simulink subsystem "calcErrorOuterLoop"  (R2026a)
settings: Solver=VariableStepAuto
settings Model: Creator=maxhu  LastModifiedBy=maxhu

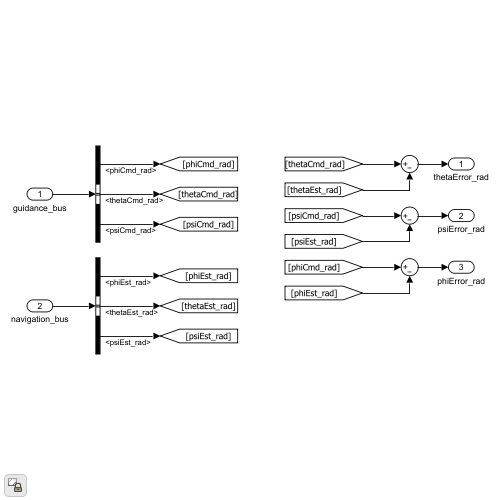
[thumbnail: Simulink's stored preview of the top-level diagram]
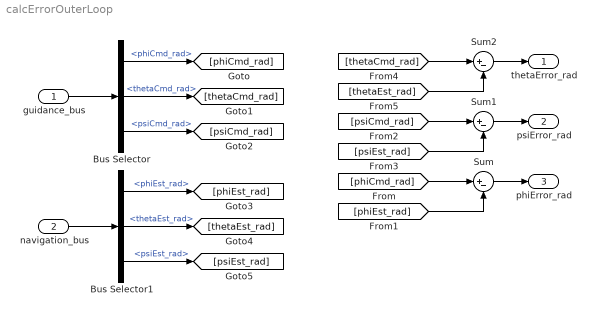
== system calcErrorOuterLoop ==
  guidance_bus : Inport
  navigation_bus : Inport  Port=2
  Bus Selector : BusSelector  OutputSignals=phiCmd_rad,thetaCmd_rad,psiCmd_rad
  Bus Selector1 : BusSelector  OutputSignals=phiEst_rad,thetaEst_rad,psiEst_rad
  Sum : Sum  Inputs=|+-
  Sum1 : Sum  Inputs=|+-
  Sum2 : Sum  Inputs=|+-
  thetaError_rad : Outport
  psiError_rad : Outport  Port=2
  phiError_rad : Outport  Port=3
  wires:
  guidance_bus/1 -> Bus Selector/1
  Bus Selector/1 -> [phiCmd_rad]  "<phiCmd_rad>"
  Bus Selector/2 -> [thetaCmd_rad]  "<thetaCmd_rad>"
  Bus Selector/3 -> [psiCmd_rad]  "<psiCmd_rad>"
  navigation_bus/1 -> Bus Selector1/1
  Bus Selector1/1 -> [phiEst_rad]  "<phiEst_rad>"
  Bus Selector1/2 -> [thetaEst_rad]  "<thetaEst_rad>"
  Bus Selector1/3 -> [psiEst_rad]  "<psiEst_rad>"
  [phiCmd_rad] -> Sum/1
  [phiEst_rad] -> Sum/2
  Sum/1 -> phiError_rad/1
  [psiCmd_rad] -> Sum1/1
  [psiEst_rad] -> Sum1/2
  Sum1/1 -> psiError_rad/1
  [thetaCmd_rad] -> Sum2/1
  [thetaEst_rad] -> Sum2/2
  Sum2/1 -> thetaError_rad/1
